simulink model "Model"  (R2025b)
settings: Solver=VariableStepAuto  StartTime=0.0  StopTime=10  RelTol=1e-3
values from neighbouring files (symbols this model uses):
  A = [ ... (first row only)    [model_params.m]
  B = [ ... (first row only)    [model_params.m]
  C = [ ... (first row only)    [model_params.m]
  D = [ ... (first row only)    [model_params.m]
libraries: uavutilslib x1
settings Model: Creator=Max  LastModifiedBy=Max

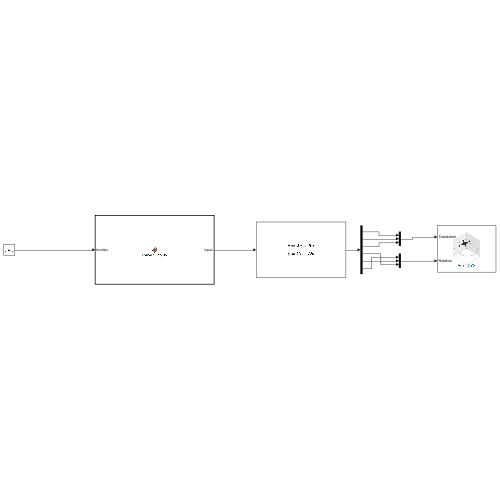
[thumbnail: Simulink's stored preview of the top-level diagram]
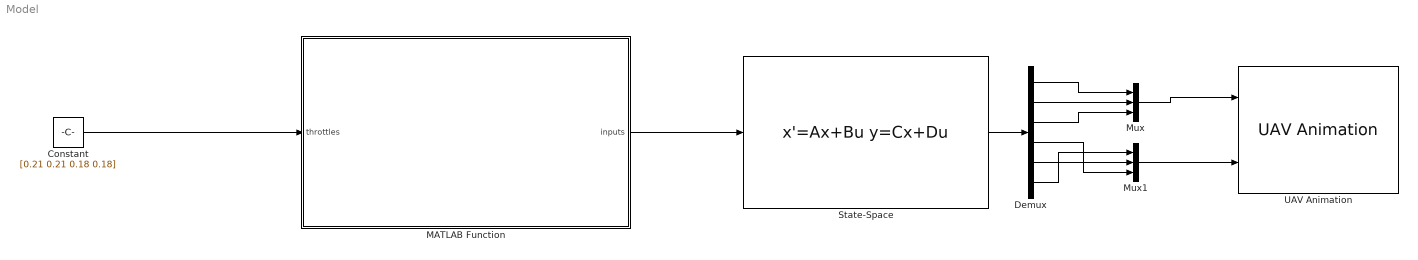
== system Model ==
  Constant : Constant  Value=[0.21 0.21 0.18 0.18]
  Demux : Demux  Outputs=6
  MATLAB Function : MATLAB Function  TreatAsAtomicUnit=on
  Mux : Mux  Inputs=3
  Mux1 : Mux  Inputs=3
  State-Space : StateSpace  A=A  B=B  C=C  D=D  InitialCondition=0
  UAV Animation : uavutilslib/UAV Animation  NumUAV=1  DynamicUAVConfig=off  UAVType=Multirotor  UAVSize=1  UAVColor=[1 0 0]  UAVTrajectoryAlpha=1  InertialZDirection=Down  RotationFormat=Euler ZYX  DrawMarkers=off  SampleTime=-1
  wires:
  MATLAB Function/1(inputs) -> State-Space/1
  State-Space/1 -> Demux/1
  Demux/1 -> Mux/1
  Demux/2 -> Mux/2
  Demux/3 -> Mux/3
  Mux/1 -> UAV Animation/1
  Demux/4 -> Mux1/3
  Demux/5 -> Mux1/2
  Mux1/1 -> UAV Animation/2
  Constant/1 -> MATLAB Function/1(throttles)
  Demux/6 -> Mux1/1

== matlab function Model/MATLAB Function ==
  data: throttles input; inputs output
function inputs = convert_inputs(throttles)
    inputs = zeros(4, 1);

    COEFFS_FORCE = [3.98646882e-04, 7.66327150e-02, -2.28383170e+00];
    COEFFS_TORQUE = [7.20894649e-06, 2.80295913e-03, -7.45248620e-02];
    DISTANCE_ROTOR_CENTER = 0.3;

    forces = polyval(COEFFS_FORCE, throttles);
    torque = polyval(COEFFS_TORQUE, throttles);

    inputs(1) = sum(forces); % thrust
    inputs(2) = DISTANCE_ROTOR_CENTER * (forces(1) - forces(2) - forces(3) + forces(4)); % roll_torque
    inputs(3) = DISTANCE_ROTOR_CENTER * (forces(1) - forces(3) + forces(2) - forces(4)); % pitch_torque
    
    
    inputs(4) = torque(1) - torque(2) + torque(3) - torque(4); % yaw torque
end
